simulink model "Ejercicio_3"  (R2021b)
settings: Solver=VariableStepAuto  StartTime=0.0  StopTime=10.0  RelTol=1e-3
libraries: commrandsrc3 x1
settings Model: Creator=Hagui  LastModifiedBy=Hagui

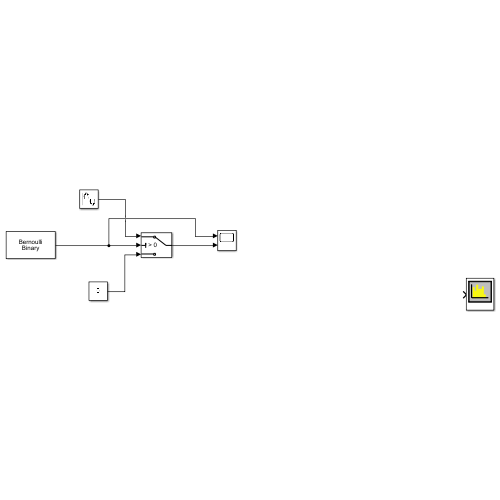
[thumbnail: Simulink's stored preview of the top-level diagram]
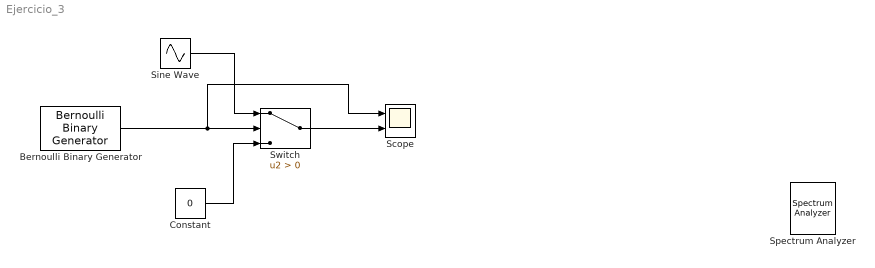
== system Ejercicio_3 ==
  Bernoulli Binary Generator : commrandsrc3/Bernoulli Binary Generator  ProbabilityOfZero=0.5  SeedSource=Auto  Seed=0  SampleTime=1  SamplesPerFrame=1  OutputDataType=double  SimulateUsing=Interpreted execution
  Constant : Constant  Value=0
  Scope : Scope  NumInputPorts=2
  Sine Wave : Sin  Frequency=4*pi*100  SampleTime=0.0001
  Spectrum Analyzer : SpectrumAnalyzer
  Switch : Switch  Criteria=u2 > Threshold
  wires:
  Bernoulli Binary Generator/1 -> Scope/1, Switch/2
  Sine Wave/1 -> Switch/1
  Constant/1 -> Switch/3
  Switch/1 -> Scope/2
